simulink model "Lab5_2"  (R2021a)
settings: Solver=ode45  StartTime=0.0  StopTime=3  RelTol=1e-3
values from neighbouring files (symbols this model uses):
  degs2rpm = 60/360    (= 0.166666666667)    [VarLab5.m]
  delta = 1/sqrt(2)    [VarLab5.m]
  Ki = 4.0    (= 4)    [VarLab5.m]
  KpP = 1    [VarLab5.m]
  KpPI = 0.01    [VarLab5.m]
  N = 10    [VarLab5.m]
  omegac = 2*pi*50    (= 314.159265359)    [VarLab5.m]
  rads2rpm = 60/2/pi    (= 9.54929658551)    [VarLab5.m]
  rpm2rads = 2*pi/60    (= 0.10471975512)    [VarLab5.m]
  Tc = 1/(2*pi*50)    (= 0.00318309886184)    [VarLab5.m]
  Ts = 1e-3    (= 0.001)    [VarLab5.m]
undefined symbols (not defined in the file or in its folder): daq, drv, gbox, mld, mot, sens
settings Model: Creator=bonvoltnuovo  LastModifiedBy=bonvoltnuovo
settings SolverCC: ZeroCrossAlgorithm=Adaptive
settings DebuggingCC: IgnoredZcDiagnostic=none

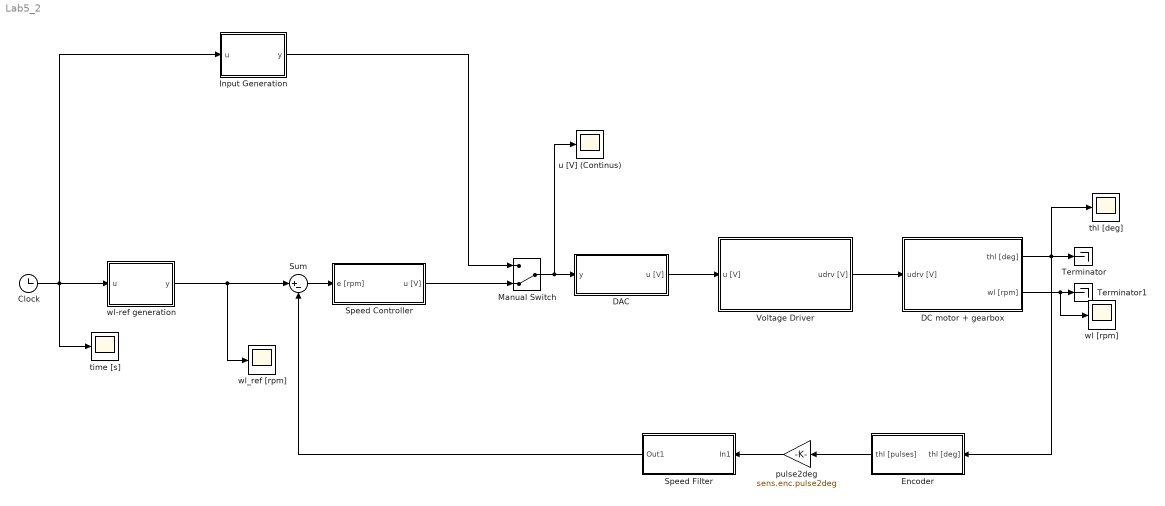
== system Lab5_2 ==
  Clock : Clock
  DAC : Subsystem
  DC motor + gearbox : Subsystem
  Encoder : Subsystem
  Input Generation : MATLAB Function  TreatAsAtomicUnit=on
  Manual Switch : ManualSwitch  CurrentSetting=0
  Speed Controller : Subsystem
  Speed Filter : Subsystem
  Sum : Sum  Inputs=|+-
  Terminator : Terminator
  Terminator1 : Terminator
  Voltage Driver : Subsystem
  pulse2deg : Gain  Gain=sens.enc.pulse2deg
  thl [deg] : Scope
  time [s] : Scope
  u [V] (Continus) : Scope
  wl [rpm] : Scope
  wl-ref generation : MATLAB Function  TreatAsAtomicUnit=on
  wl_ref [rpm] : Scope
  wires:
  DAC/1(u [V]) -> Voltage Driver/1(u [V])
  Voltage Driver/1(udrv [V]) -> DC motor + gearbox/1(udrv [V])
  DC motor + gearbox/2(wl [rpm]) -> wl [rpm]/1, Terminator1/1
  DC motor + gearbox/1(thl [deg]) -> thl [deg]/1, Terminator/1, Encoder/1(thl [deg])
  pulse2deg/1 -> Speed Filter/1(In1)
  Encoder/1(thl [pulses]) -> pulse2deg/1
  Speed Filter/1(Out1) -> Sum/2
  wl-ref generation/1(y) -> Sum/1, wl_ref [rpm]/1
  Sum/1 -> Speed Controller/1(e [rpm])
  Clock/1 -> Input Generation/1(u), wl-ref generation/1(u), time [s]/1
  Input Generation/1(y) -> Manual Switch/1
  Manual Switch/1 -> u [V] (Continus)/1, DAC/1(y)
  Speed Controller/1(u [V]) -> Manual Switch/2

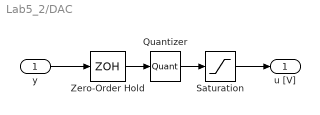
== system Lab5_2/DAC ==
  y : Inport
  Quantizer : Quantizer  QuantizationInterval=daq.dac.q
  Saturation : Saturate  UpperLimit=daq.dac.fs  LowerLimit=-1*daq.dac.fs
  Zero-Order Hold : ZeroOrderHold  SampleTime=Ts
  u [V] : Outport
  wires:
  y/1 -> Zero-Order Hold/1
  Zero-Order Hold/1 -> Quantizer/1
  Quantizer/1 -> Saturation/1
  Saturation/1 -> u [V]/1

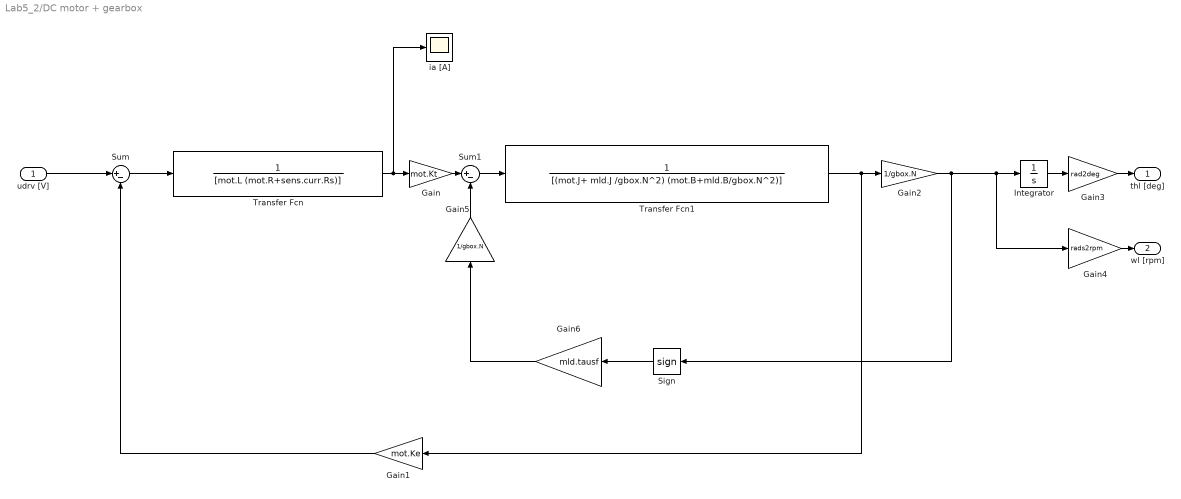
== system Lab5_2/DC motor + gearbox ==
  udrv [V] : Inport
  Gain : Gain  Gain=mot.Kt
  Gain1 : Gain  Gain=mot.Ke
  Gain2 : Gain  Gain=1/gbox.N
  Gain3 : Gain  Gain=rad2deg
  Gain4 : Gain  Gain=rads2rpm
  Gain5 : Gain  Gain=1/gbox.N
  Gain6 : Gain  Gain=mld.tausf
  Integrator : Integrator
  Sign : Signum  ZeroCross=off
  Sum : Sum  Inputs=|+-
  Sum1 : Sum  Inputs=|+-
  Transfer Fcn : TransferFcn  Denominator=[mot.L (mot.R+sens.curr.Rs)]
  Transfer Fcn1 : TransferFcn  Denominator=[(mot.J+ mld.J /gbox.N^2) (mot.B+mld.B/gbox.N^2)]
  ia [A] : Scope
  thl [deg] : Outport
  wl [rpm] : Outport  Port=2
  wires:
  udrv [V]/1 -> Sum/1
  Gain/1 -> Sum1/1
  Transfer Fcn/1 -> ia [A]/1, Gain/1
  Sum/1 -> Transfer Fcn/1
  Sum1/1 -> Transfer Fcn1/1
  Transfer Fcn1/1 -> Gain1/1, Gain2/1
  Gain2/1 -> Gain4/1, Integrator/1, Sign/1
  Integrator/1 -> Gain3/1
  Gain3/1 -> thl [deg]/1
  Gain4/1 -> wl [rpm]/1
  Gain1/1 -> Sum/2
  Gain5/1 -> Sum1/2
  Sign/1 -> Gain6/1
  Gain6/1 -> Gain5/1

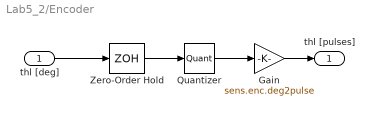
== system Lab5_2/Encoder ==
  thl [deg] : Inport
  Gain : Gain  Gain=sens.enc.deg2pulse
  Quantizer : Quantizer  QuantizationInterval=sens.enc.pulse2deg
  Zero-Order Hold : ZeroOrderHold  SampleTime=Ts
  thl [pulses] : Outport
  wires:
  Zero-Order Hold/1 -> Quantizer/1
  Gain/1 -> thl [pulses]/1
  thl [deg]/1 -> Zero-Order Hold/1
  Quantizer/1 -> Gain/1

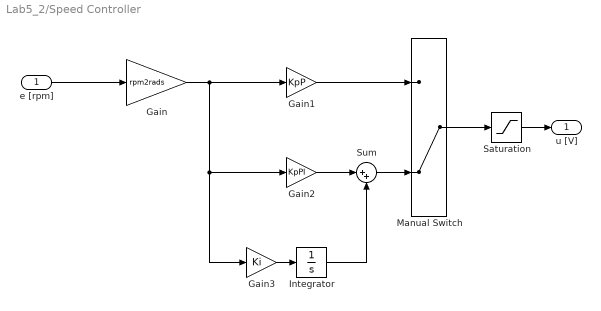
== system Lab5_2/Speed Controller ==
  e [rpm] : Inport
  Gain : Gain  Gain=rpm2rads
  Gain1 : Gain  Gain=KpP
  Gain2 : Gain  Gain=KpPI
  Gain3 : Gain  Gain=Ki
  Integrator : Integrator
  Manual Switch : ManualSwitch  CurrentSetting=0
  Saturation : Saturate  UpperLimit=20  LowerLimit=-20
  Sum : Sum  Inputs=|++
  u [V] : Outport
  wires:
  Gain/1 -> Gain3/1, Gain2/1, Gain1/1
  e [rpm]/1 -> Gain/1
  Gain1/1 -> Manual Switch/1
  Gain3/1 -> Integrator/1
  Manual Switch/1 -> Saturation/1
  Saturation/1 -> u [V]/1
  Integrator/1 -> Sum/2
  Sum/1 -> Manual Switch/2
  Gain2/1 -> Sum/1

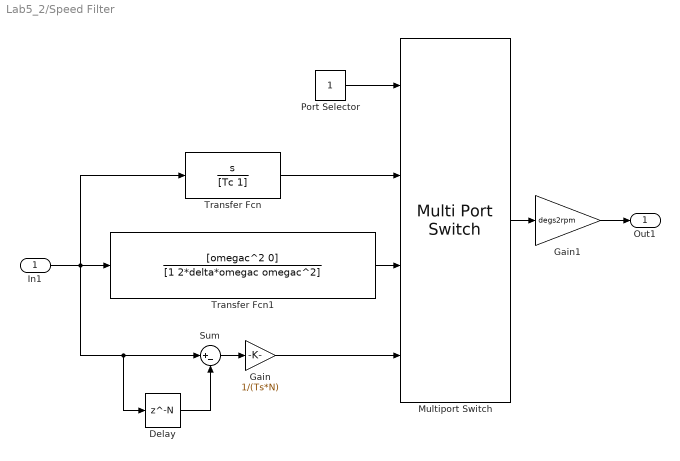
== system Lab5_2/Speed Filter ==
  In1 : Inport
  Delay : Delay  DelayLength=N
  Gain : Gain  Gain=1/(Ts*N)
  Gain1 : Gain  Gain=degs2rpm
  Multiport Switch : MultiPortSwitch
  Port Selector : Constant
  Sum : Sum  Inputs=|+-
  Transfer Fcn : TransferFcn  Numerator=[1 0]  Denominator=[Tc 1]
  Transfer Fcn1 : TransferFcn  Numerator=[omegac^2 0]  Denominator=[1 2*delta*omegac omegac^2]
  Out1 : Outport
  wires:
  Transfer Fcn/1 -> Multiport Switch/2
  Port Selector/1 -> Multiport Switch/1
  Multiport Switch/1 -> Gain1/1
  Gain1/1 -> Out1/1
  In1/1 -> Delay/1, Sum/1, Transfer Fcn/1, Transfer Fcn1/1
  Transfer Fcn1/1 -> Multiport Switch/3
  Sum/1 -> Gain/1
  Delay/1 -> Sum/2
  Gain/1 -> Multiport Switch/4

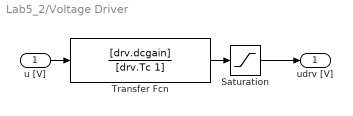
== system Lab5_2/Voltage Driver ==
  u [V] : Inport
  Saturation : Saturate  UpperLimit=drv.outmax  LowerLimit=-1*drv.outmax
  Transfer Fcn : TransferFcn  Numerator=[drv.dcgain]  Denominator=[drv.Tc 1]
  udrv [V] : Outport
  wires:
  Saturation/1 -> udrv [V]/1
  u [V]/1 -> Transfer Fcn/1
  Transfer Fcn/1 -> Saturation/1

== matlab function Lab5_2/wl-ref generation ==
  data: u input; y output
function y = fcn(u)
    y=0;
    if(u>=0 && u<1.5)
        y=250;
    end
    if(u>=1.5 && u<3)
        y=-250;
    end
end

== matlab function Lab5_2/Input Generation ==
  data: u input; y output
function y = fcn(u)
    y=0;
    if(u>=0 && u<1.5)
        y=6;
    end
    if(u>=1.5 && u<3)
        y=-6;
    end
end
